simulink model "NLvsTF"  (R2020b)
settings: Solver=VariableStepAuto  StartTime=0.0  StopTime=10  RelTol=1e-3
values from neighbouring files (symbols this model uses):
  alfa_r = (alfa_g*pi)/180    (= -0.460854188989)    [params.m]
  Fpv = p2*alfa_v^2+p1*alfa_v+p0    (= 0.1075)    [params.m]
  g = 9.81    [params.m]
  I = m1*r1^2+m2*r2^2+m3*r3^2    (= 0.0018475)    [params.m]
  kf = a2*-1.4249^2+a0    (= 0.00161666870055)    [params.m]
  m1 = 0.031    [params.m]
  r1 = 0.19    [params.m]
settings Model: Creator=bou  LastModifiedBy=bou
settings SolverCC: AlgebraicLoopSolver=LineSearch

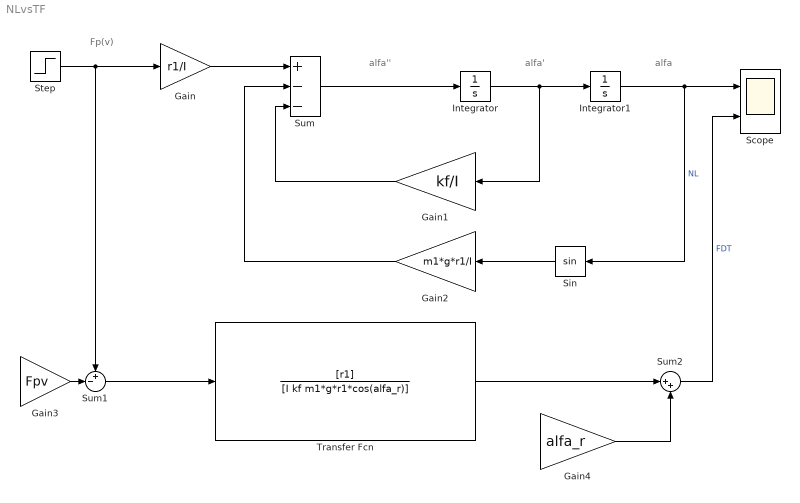
== system NLvsTF ==
  note: Fp(v)
  note: alfa
  note: alfa'
  note: alfa''
  Gain : Gain  Gain=r1/I
  Gain1 : Gain  Gain=kf/I
  Gain2 : Gain  Gain=m1*g*r1/I
  Gain3 : Gain  Gain=Fpv
  Gain4 : Gain  Gain=alfa_r
  Integrator : Integrator  InitialCondition=m1*g*sin(alfa_r)
  Integrator1 : Integrator  InitialCondition=m1*g*sin(alfa_r)
  Scope : Scope  NumInputPorts=2
  Sin : Trigonometry
  Step : Step  Time=0  Before=m1*g*sin(alfa_r)  After=m1*g*sin(alfa_r)  SampleTime=0
  Sum : Sum  Inputs=+--
  Sum1 : Sum  Inputs=+-|
  Sum2 : Sum  Inputs=|++
  Transfer Fcn : TransferFcn  Numerator=[r1]  Denominator=[I kf m1*g*r1*cos(alfa_r)]
  wires:
  Integrator1/1 -> Sin/1, Scope/1  "NL"
  Integrator/1 -> Gain1/1, Integrator1/1
  Sum/1 -> Integrator/1
  Gain/1 -> Sum/1
  Gain1/1 -> Sum/3
  Gain2/1 -> Sum/2
  Sin/1 -> Gain2/1
  Step/1 -> Sum1/1, Gain/1
  Gain3/1 -> Sum1/2
  Sum1/1 -> Transfer Fcn/1
  Transfer Fcn/1 -> Sum2/1
  Sum2/1 -> Scope/2  "FDT"
  Gain4/1 -> Sum2/2
